simulink model "new68bus_opal"  (R2019b)
settings: Solver=ode4  StartTime=0.0  StopTime=30  FixedStep=Ts  RelTol=1e-3
PreLoadFcn:
  | PSSMODEL=1;
  | LPSS=0;
  | WAPSS=0;
  | WAPSS2=0;
  | Ts=50e-5;
InitFcn:
  | PSSMODEL=1;
  | LPSS=0;
  | WAPSS=0;
  | WAPSS2=0;
  | Ts=50e-5;
  | 
  | % Required data to 68 Bus benchmark
  | % clear
  | % clc
  | % Definition for the columns
  | % system base =100 MVA
  | 
  | %% Line data Format (line)
  | % All values are given on the same system base MVA
  | % 1: From bus
  | % 2: To bus
  | % 3: Resistance (pu)
  | % 4: Reactance  (pu)
  | % 5: Charge     (pu)
  | % 6: Transformer Tap Amplitute
  | % 7: base MVA
  | % 8: Nomonal Voltage (KV)
  | 
  | %1   2    3        4       5       6        7      8
  | line=[...
  | 1	54	0	     0.0181	  0	      1.025     100    13.8
  | 2	58	0	     0.025	  0	      1.070     100    13.8
  | 3	62	0	     0.02	  0	      1.070     100    13.8
  | 4	19	0.0007	 0.0142	  0	      1.070     100    13.8
  | 5	20	0.0009	 0.018	  0	      1.009     100    13.8
  | 6	22	0	     0.0143	  0	      1.025     100    13.8
  | 7	23	0.0005	 0.0272	  0	      0         100    13.8
  | 8	25	0.0006	 0.0232	  0	      1.025     100    13.8
  | 9	29	0.0008	 0.0156   0	      1.025     100    13.8
  | 10	31	0	     0.026	  0	      1.04      100    13.8
  | 11	32	0	     0.013	  0	      1.04      100    13.8
  | 12	36	0	     0.0075	  0	      1.04      100    13.8
  | 13	17	0	     0.0033	  0	      1.04      100    13.8
  | 14	41	0	     0.0015	  0	      1         100    13.8
  | 15	42	0	     0.0015	  0	      1         100    13.8
  | 16	18	0	     0.003	  0	      1         100    13.8
  | 17	36	0.0005	 0.0045	  0.32	  0         100    138
  | 17	43	0.0005	 0.0276	  0	      0         100    138
  | 18	42	0.004	 0.06	  2.25    0         100    138
  | 18	49	0.0076	 0.1141	  1.16    0	        100    138
  | 18	50	0.0012	 0.0288	  2.06	  0         100    138
  | 20	19	0.0007	 0.0138	  0       1.06	    100    138
  | 19	68	0.0016	 0.0195	  0.304	  0         100    138
  | 21	22	0.0008	 0.014	  0.2565  0	        100    138
  | 21	68	0.0008	 0.0135	  0.2548  0	        100    138
  | 22	23	0.0006	 0.0096	  0.1846  0	        100    138
  | 23	24	0.0022	 0.035	  0.361	  0         100    138
  | 24	68	0.0003	 0.0059	  0.068	  0         100    138
  | 25	26	0.0032	 0.0323	  0.531	  0         100    138
  | 25	54	0.007	 0.0086	  0.146	  0         100    138
  | 26	27	0.0014	 0.0147	  0.2396  0	        100    138
  | 26	28	0.0043	 0.0474	  0.7802  0	        100    138
  | 26	29	0.0057	 0.0625	  1.029	  0         100    138
  | 27	37	0.0013	 0.0173	  0.3216  0	        100    138
  | 27	53	0.032	 0.32	  0.41	  0         100    138
  | ... (+206 lines)
undefined symbols (not defined in the file or in its folder): D1, Delta, I, Left, Right, type, V
libraries: powerlib x359, artemis x26, sps_avr x16, powerlib_meascontrol x5, rtlab x1
(part 5 of 8)

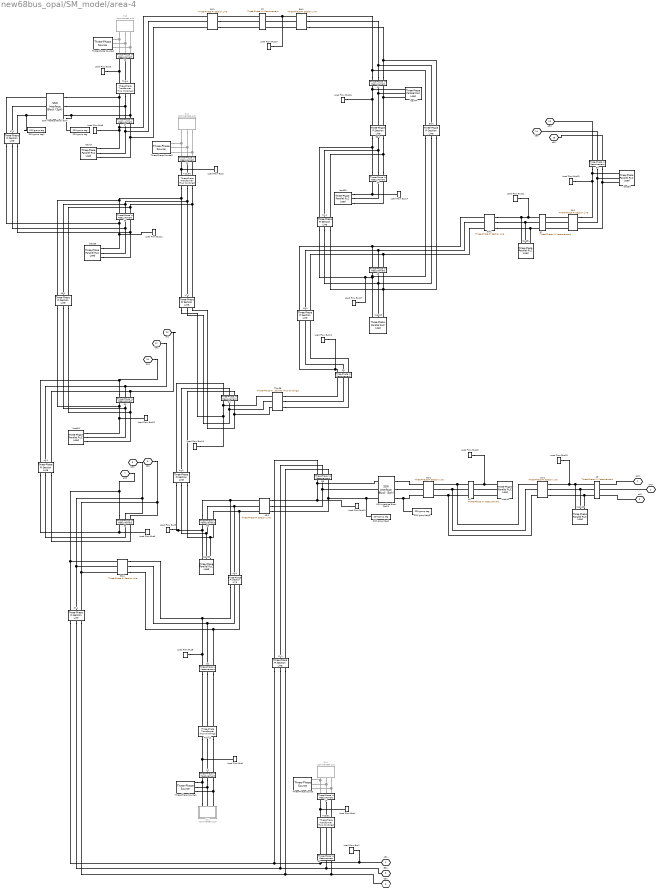
== system new68bus_opal/SM_model/area-4 ==
  10 : powerlib/Measurements/Three-Phase V-I Measurement  VoltageMeasurement=phase-to-phase  SetLabelV=on  LabelV=Vabc_10  Vpu=off  VpuLL=on  CurrentMeasurement=no  SetLabelI=off  LabelI=Iabc  Ipu=off  Pbase=100e6  Vbase=13.8e3  OutputType=Complex  PhasorSimulation=off  PSBequivalent=0
      settings: SourceProductName=Simscape Electrical
  11 : powerlib/Measurements/Three-Phase V-I Measurement  VoltageMeasurement=phase-to-phase  SetLabelV=on  LabelV=Vabc_11  Vpu=off  VpuLL=on  CurrentMeasurement=no  SetLabelI=off  LabelI=Iabc  Ipu=off  Pbase=100e6  Vbase=13.8e3  OutputType=Complex  PhasorSimulation=off  PSBequivalent=0
      settings: SourceProductName=Simscape Electrical
  12 : powerlib/Measurements/Three-Phase V-I Measurement  VoltageMeasurement=phase-to-phase  SetLabelV=on  LabelV=Vabc_12  Vpu=off  VpuLL=on  CurrentMeasurement=no  SetLabelI=off  LabelI=Iabc  Ipu=off  Pbase=100e6  Vbase=13.8e3  OutputType=Complex  PhasorSimulation=off  PSBequivalent=0
      settings: SourceProductName=Simscape Electrical
  13 : powerlib/Measurements/Three-Phase V-I Measurement  VoltageMeasurement=phase-to-phase  SetLabelV=on  LabelV=Vabc_13  Vpu=off  VpuLL=on  CurrentMeasurement=no  SetLabelI=off  LabelI=Iabc  Ipu=off  Pbase=100e6  Vbase=13.8e3  OutputType=Complex  PhasorSimulation=off  PSBequivalent=0
      settings: SourceProductName=Simscape Electrical
  17 : powerlib/Measurements/Three-Phase V-I Measurement  VoltageMeasurement=phase-to-phase  SetLabelV=on  LabelV=Vabc_17  Vpu=off  VpuLL=on  CurrentMeasurement=no  SetLabelI=off  LabelI=Iabc  Ipu=off  Pbase=100e6  Vbase=Bus(17,2)*1e3  OutputType=Complex  PhasorSimulation=off  PSBequivalent=0
      settings: SourceProductName=Simscape Electrical
  17-1 : powerlib/Elements/Three-Phase PI Section Line  LConnTagsString=a|b|c  RConnTagsString=A|B|C  Frequency=60  Resistances=[line(17,3) 3*line(17,3)]  Inductances=[line(17,4) 3*line(17,4)]  Capacitances=[line(17,5) line(17,5)/3]  Length=1
      settings: SourceProductName=Simscape Electrical
  18-1 : powerlib/Elements/Three-Phase PI Section Line  LConnTagsString=a|b|c  RConnTagsString=A|B|C  Frequency=60  Resistances=[line(18,3) 3*line(18,3)]  Inductances=[line(18,4) 3*line(18,4)]  Capacitances=[line(28,5) line(28,5)/3]  Length=1
      settings: SourceProductName=Simscape Electrical
  30 : powerlib/Measurements/Three-Phase V-I Measurement  VoltageMeasurement=phase-to-phase  SetLabelV=on  LabelV=Vabc_30  Vpu=off  VpuLL=on  CurrentMeasurement=no  SetLabelI=off  LabelI=Iabc  Ipu=off  Pbase=100e6  Vbase=Bus(30,2)*1e3  OutputType=Complex  PhasorSimulation=off  PSBequivalent=0
      settings: SourceProductName=Simscape Electrical
  31 : powerlib/Measurements/Three-Phase V-I Measurement  VoltageMeasurement=phase-to-phase  SetLabelV=on  LabelV=Vabc_31  Vpu=off  VpuLL=on  CurrentMeasurement=no  SetLabelI=off  LabelI=Iabc  Ipu=off  Pbase=100e6  Vbase=Bus(31,2)*1e3  OutputType=Complex  PhasorSimulation=off  PSBequivalent=0
      settings: SourceProductName=Simscape Electrical
  32 : powerlib/Measurements/Three-Phase V-I Measurement  VoltageMeasurement=phase-to-phase  SetLabelV=on  LabelV=Vabc_32  Vpu=off  VpuLL=on  CurrentMeasurement=no  SetLabelI=off  LabelI=Iabc  Ipu=off  Pbase=100e6  Vbase=Bus(32,2)*1e3  OutputType=Complex  PhasorSimulation=off  PSBequivalent=0
      settings: SourceProductName=Simscape Electrical
  33 : powerlib/Measurements/Three-Phase V-I Measurement  VoltageMeasurement=phase-to-phase  SetLabelV=on  LabelV=Vabc_33  Vpu=off  VpuLL=on  CurrentMeasurement=no  SetLabelI=off  LabelI=Iabc  Ipu=off  Pbase=100e6  Vbase=Bus(33,2)*1e3  OutputType=Complex  PhasorSimulation=off  PSBequivalent=0
      settings: SourceProductName=Simscape Electrical
  34 : powerlib/Measurements/Three-Phase V-I Measurement  VoltageMeasurement=phase-to-phase  SetLabelV=on  LabelV=Vabc_34  Vpu=off  VpuLL=on  CurrentMeasurement=no  SetLabelI=off  LabelI=Iabc  Ipu=off  Pbase=100e6  Vbase=Bus(34,2)*1e3  OutputType=Complex  PhasorSimulation=off  PSBequivalent=0
      settings: SourceProductName=Simscape Electrical
  35 : powerlib/Measurements/Three-Phase V-I Measurement  VoltageMeasurement=phase-to-phase  SetLabelV=on  LabelV=Vabc_35  Vpu=off  VpuLL=on  CurrentMeasurement=no  SetLabelI=off  LabelI=Iabc  Ipu=off  Pbase=100e6  Vbase=Bus(35,2)*1e3  OutputType=Complex  PhasorSimulation=off  PSBequivalent=0
      settings: SourceProductName=Simscape Electrical
  36 : powerlib/Measurements/Three-Phase V-I Measurement  VoltageMeasurement=phase-to-phase  SetLabelV=on  LabelV=Vabc_36  Vpu=off  VpuLL=on  CurrentMeasurement=no  SetLabelI=off  LabelI=Iabc  Ipu=off  Pbase=100e6  Vbase=Bus(36,2)*1e3  OutputType=Complex  PhasorSimulation=off  PSBequivalent=0
      settings: SourceProductName=Simscape Electrical
  37-1 : powerlib/Elements/Three-Phase PI Section Line  LConnTagsString=a|b|c  RConnTagsString=A|B|C  Frequency=60  Resistances=[line(37,3) 3*line(37,3)]  Inductances=[line(37,4) 3*line(37,4)]  Capacitances=[line(37,5) line(37,5)/3]  Length=1
      settings: SourceProductName=Simscape Electrical
  38 : powerlib/Measurements/Three-Phase V-I Measurement  VoltageMeasurement=phase-to-phase  SetLabelV=on  LabelV=Vabc_38  Vpu=off  VpuLL=on  CurrentMeasurement=no  SetLabelI=off  LabelI=Iabc  Ipu=off  Pbase=100e6  Vbase=Bus(38,2)*1e3  OutputType=Complex  PhasorSimulation=off  PSBequivalent=0
      settings: SourceProductName=Simscape Electrical
  38-1 : powerlib/Elements/Three-Phase PI Section Line  LConnTagsString=a|b|c  RConnTagsString=A|B|C  Frequency=60  Resistances=[line(38,3) 3*line(38,3)]  Inductances=[line(38,4) 3*line(38,4)]  Capacitances=[line(38,5) line(38,5)/3]  Length=1
      settings: SourceProductName=Simscape Electrical
  39 : powerlib/Measurements/Three-Phase V-I Measurement  VoltageMeasurement=phase-to-phase  SetLabelV=on  LabelV=Vabc_39  Vpu=off  VpuLL=on  CurrentMeasurement=no  SetLabelI=off  LabelI=Iabc  Ipu=off  Pbase=100e6  Vbase=Bus(39,2)*1e3  OutputType=Complex  PhasorSimulation=off  PSBequivalent=0
      settings: SourceProductName=Simscape Electrical
  40-1 : powerlib/Elements/Three-Phase PI Section Line  LConnTagsString=a|b|c  RConnTagsString=A|B|C  Frequency=60  Resistances=[line(40,3) 3*line(40,3)]  Inductances=[line(40,4) 3*line(40,4)]  Capacitances=[line(40,5) line(40,5)/3]  Length=1
      settings: SourceProductName=Simscape Electrical
  41-1 : powerlib/Elements/Three-Phase PI Section Line  LConnTagsString=a|b|c  RConnTagsString=A|B|C  Frequency=60  Resistances=[line(45,3) 3*line(45,3)]  Inductances=[line(45,4) 3*line(45,4)]  Capacitances=[line(45,5) line(45,5)/3]  Length=1
      settings: SourceProductName=Simscape Electrical
  43 : powerlib/Measurements/Three-Phase V-I Measurement  VoltageMeasurement=phase-to-phase  SetLabelV=on  LabelV=Vabc_43  Vpu=off  VpuLL=on  CurrentMeasurement=no  SetLabelI=off  LabelI=Iabc  Ipu=off  Pbase=100e6  Vbase=Bus(43,2)*1e3  OutputType=Complex  PhasorSimulation=off  PSBequivalent=0
      settings: SourceProductName=Simscape Electrical
  43-1 : powerlib/Elements/Three-Phase PI Section Line  LConnTagsString=a|b|c  RConnTagsString=A|B|C  Frequency=60  Resistances=[line(43,3) 3*line(43,3)]  Inductances=[line(43,4) 3*line(43,4)]  Capacitances=[line(43,5) line(43,5)/3]  Length=1
      settings: SourceProductName=Simscape Electrical
  44 : powerlib/Measurements/Three-Phase V-I Measurement  VoltageMeasurement=phase-to-phase  SetLabelV=on  LabelV=Vabc_44  Vpu=off  VpuLL=on  CurrentMeasurement=no  SetLabelI=off  LabelI=Iabc  Ipu=off  Pbase=100e6  Vbase=Bus(44,2)*1e3  OutputType=Complex  PhasorSimulation=off  PSBequivalent=0
      settings: SourceProductName=Simscape Electrical
  44-1 : powerlib/Elements/Three-Phase PI Section Line  LConnTagsString=a|b|c  RConnTagsString=A|B|C  Frequency=60  Resistances=[line(44,3) 3*line(44,3)]  Inductances=[line(44,4) 3*line(44,4)]  Capacitances=[line(44,5) line(44,5)/3]  Length=1
      settings: SourceProductName=Simscape Electrical
  45 : powerlib/Measurements/Three-Phase V-I Measurement  VoltageMeasurement=phase-to-phase  SetLabelV=on  LabelV=Vabc_45  Vpu=off  VpuLL=on  CurrentMeasurement=no  SetLabelI=off  LabelI=Iabc  Ipu=off  Pbase=100e6  Vbase=Bus(45,2)*1e3  OutputType=Complex  PhasorSimulation=off  PSBequivalent=0
      settings: SourceProductName=Simscape Electrical
  45-1 : powerlib/Elements/Three-Phase PI Section Line  LConnTagsString=a|b|c  RConnTagsString=A|B|C  Frequency=60  Resistances=[line(45,3) 3*line(45,3)]  Inductances=[line(45,4) 3*line(45,4)]  Capacitances=[line(45,5) line(45,5)/3]  Length=1
      settings: SourceProductName=Simscape Electrical
  46 : powerlib/Measurements/Three-Phase V-I Measurement  VoltageMeasurement=phase-to-phase  SetLabelV=on  LabelV=Vabc_46  Vpu=off  VpuLL=on  CurrentMeasurement=no  SetLabelI=off  LabelI=Iabc  Ipu=off  Pbase=100e6  Vbase=Bus(46,2)*1e3  OutputType=Complex  PhasorSimulation=off  PSBequivalent=0
      settings: SourceProductName=Simscape Electrical
  47-1 : powerlib/Elements/Three-Phase PI Section Line  LConnTagsString=a|b|c  RConnTagsString=A|B|C  Frequency=60  Resistances=[line(47,3) 3*line(47,3)]  Inductances=[line(47,4) 3*line(47,4)]  Capacitances=[line(47,5) line(47,5)/3]  Length=1
      settings: SourceProductName=Simscape Electrical
  48-1 : powerlib/Elements/Three-Phase PI Section Line  LConnTagsString=a|b|c  RConnTagsString=A|B|C  Frequency=60  Resistances=[line(48,3) 3*line(48,3)]  Inductances=[line(48,4) 3*line(48,4)]  Capacitances=[line(48,5) line(48,5)/3]  Length=1
      settings: SourceProductName=Simscape Electrical
  49 : powerlib/Measurements/Three-Phase V-I Measurement  VoltageMeasurement=phase-to-phase  SetLabelV=on  LabelV=Vabc_49  Vpu=off  VpuLL=on  CurrentMeasurement=no  SetLabelI=off  LabelI=Iabc  Ipu=off  Pbase=100e6  Vbase=Bus(49,2)*1e3  OutputType=Complex  PhasorSimulation=off  PSBequivalent=0
      settings: SourceProductName=Simscape Electrical
  49-1 : powerlib/Elements/Three-Phase PI Section Line  LConnTagsString=a|b|c  RConnTagsString=A|B|C  Frequency=60  Resistances=[line(49,3) 3*line(49,3)]  Inductances=[line(49,4) 3*line(49,4)]  Capacitances=[line(49,5) line(49,5)/3]  Length=1
      settings: SourceProductName=Simscape Electrical
  50 : powerlib/Measurements/Three-Phase V-I Measurement  VoltageMeasurement=phase-to-phase  SetLabelV=on  LabelV=Vabc_50  Vpu=off  VpuLL=on  CurrentMeasurement=no  SetLabelI=off  LabelI=Iabc  Ipu=off  Pbase=100e6  Vbase=Bus(50,2)*1e3  OutputType=Complex  PhasorSimulation=off  PSBequivalent=0
      settings: SourceProductName=Simscape Electrical
  51 : powerlib/Measurements/Three-Phase V-I Measurement  VoltageMeasurement=phase-to-phase  SetLabelV=on  LabelV=Vabc_51  Vpu=off  VpuLL=on  CurrentMeasurement=no  SetLabelI=off  LabelI=Iabc  Ipu=off  Pbase=100e6  Vbase=Bus(51,2)*1e3  OutputType=Complex  PhasorSimulation=off  PSBequivalent=0
      settings: SourceProductName=Simscape Electrical
  52-1 : powerlib/Elements/Three-Phase PI Section Line  LConnTagsString=a|b|c  RConnTagsString=A|B|C  Frequency=60  Resistances=[line(52,3) 3*line(52,3)]  Inductances=[line(52,4) 3*line(52,4)]  Capacitances=[line(52,5) line(52,5)/3]  Length=1
      settings: SourceProductName=Simscape Electrical
  53-1 : powerlib/Elements/Three-Phase PI Section Line  LConnTagsString=a|b|c  RConnTagsString=A|B|C  Frequency=60  Resistances=[line(52,4) 3*line(52,4)]  Inductances=[line(53,4) 3*line(53,4)]  Capacitances=[line(28,5) line(28,5)/3]  Length=1
      settings: SourceProductName=Simscape Electrical
  54-1 : powerlib/Elements/Three-Phase PI Section Line  LConnTagsString=a|b|c  RConnTagsString=A|B|C  Frequency=60  Resistances=[line(52,4) 3*line(52,4)]  Inductances=[line(54,4) 3*line(54,4)]  Capacitances=[line(28,5) line(28,5)/3]  Length=1
      settings: SourceProductName=Simscape Electrical
  58-1 : powerlib/Elements/Three-Phase PI Section Line  LConnTagsString=a|b|c  RConnTagsString=A|B|C  Frequency=60  Resistances=[line(58,3) 3*line(58,3)]  Inductances=[line(58,4) 3*line(58,4)]  Capacitances=[line(28,5) line(28,5)/3]  Length=1
      settings: SourceProductName=Simscape Electrical
  59-1 : powerlib/Elements/Three-Phase PI Section Line  LConnTagsString=a|b|c  RConnTagsString=A|B|C  Frequency=60  Resistances=[line(59,3) 3*line(59,3)]  Inductances=[line(59,4) 3*line(59,4)]  Capacitances=[line(28,5) line(28,5)/3]  Length=1
      settings: SourceProductName=Simscape Electrical
  60-1 : powerlib/Elements/Three-Phase PI Section Line  LConnTagsString=a|b|c  RConnTagsString=A|B|C  Frequency=60  Resistances=[line(60,3) 3*line(60,3)]  Inductances=[line(60,4) 3*line(60,4)]  Capacitances=[line(60,5) line(60,5)/3]  Length=1
      settings: SourceProductName=Simscape Electrical
  61 : powerlib/Measurements/Three-Phase V-I Measurement  VoltageMeasurement=phase-to-phase  SetLabelV=on  LabelV=Vabc_61  Vpu=off  VpuLL=on  CurrentMeasurement=no  SetLabelI=off  LabelI=Iabc  Ipu=off  Pbase=100e6  Vbase=Bus(61,2)*1e3  OutputType=Complex  PhasorSimulation=off  PSBequivalent=0
      settings: SourceProductName=Simscape Electrical
  61-1 : powerlib/Elements/Three-Phase PI Section Line  LConnTagsString=a|b|c  RConnTagsString=A|B|C  Frequency=60  Resistances=[line(61,3) 3*line(61,3)]  Inductances=[line(61,4) 3*line(61,4)]  Capacitances=[line(61,5) line(61,5)/3]  Length=1
      settings: SourceProductName=Simscape Electrical
  64-1 : powerlib/Elements/Three-Phase PI Section Line  LConnTagsString=a|b|c  RConnTagsString=A|B|C  Frequency=60  Resistances=[line(64,3) 3*line(64,3)]  Inductances=[line(64,4) 3*line(64,4)]  Capacitances=[line(64,5) line(64,5)/3]  Length=1
      settings: SourceProductName=Simscape Electrical
  G10 : Subsystem  Commented=on
  G11 : Subsystem  Commented=on
  G12 : Subsystem  Commented=on
  G13 : Subsystem  Commented=on
  Load Flow Bus1 : powerlib/Measurements/Load Flow Bus  LConnTagsString=a  Phases=single  Connectors=on one side  ID=BUS_11  Vbase=13.8e3  Vref=1  Vangle=0  VLF=1  VLFb=1  VLFc=1  angleLF=0  angleLFb=0  angleLFc=0
      settings: SourceProductName=Simscape Electrical
  Load Flow Bus10 : powerlib/Measurements/Load Flow Bus  LConnTagsString=a  Phases=single  Connectors=on one side  ID=BUS_34  Vbase=138e3  Vref=1  Vangle=0  VLF=1  VLFb=1  VLFc=1  angleLF=0  angleLFb=0  angleLFc=0
      settings: SourceProductName=Simscape Electrical
  Load Flow Bus11 : powerlib/Measurements/Load Flow Bus  LConnTagsString=a  Phases=single  Connectors=on one side  ID=BUS_35  Vbase=138e3  Vref=1  Vangle=0  VLF=1  VLFb=1  VLFc=1  angleLF=0  angleLFb=0  angleLFc=0
      settings: SourceProductName=Simscape Electrical
  Load Flow Bus12 : powerlib/Measurements/Load Flow Bus  LConnTagsString=a  Phases=single  Connectors=on one side  ID=BUS_36  Vbase=138e3  Vref=1  Vangle=0  VLF=1  VLFb=1  VLFc=1  angleLF=0  angleLFb=0  angleLFc=0
      settings: SourceProductName=Simscape Electrical
  Load Flow Bus13 : powerlib/Measurements/Load Flow Bus  LConnTagsString=a  Phases=single  Connectors=on one side  ID=BUS_38  Vbase=138e3  Vref=1  Vangle=0  VLF=1  VLFb=1  VLFc=1  angleLF=0  angleLFb=0  angleLFc=0
      settings: SourceProductName=Simscape Electrical
  Load Flow Bus14 : powerlib/Measurements/Load Flow Bus  LConnTagsString=a  Phases=single  Connectors=on one side  ID=BUS_39  Vbase=138e3  Vref=1  Vangle=0  VLF=1  VLFb=1  VLFc=1  angleLF=0  angleLFb=0  angleLFc=0
      settings: SourceProductName=Simscape Electrical
  Load Flow Bus15 : powerlib/Measurements/Load Flow Bus  LConnTagsString=a  Phases=single  Connectors=on one side  ID=BUS_43  Vbase=138e3  Vref=1  Vangle=0  VLF=1  VLFb=1  VLFc=1  angleLF=0  angleLFb=0  angleLFc=0
      settings: SourceProductName=Simscape Electrical
  Load Flow Bus16 : powerlib/Measurements/Load Flow Bus  LConnTagsString=a  Phases=single  Connectors=on one side  ID=BUS_44  Vbase=138e3  Vref=1  Vangle=0  VLF=1  VLFb=1  VLFc=1  angleLF=0  angleLFb=0  angleLFc=0
      settings: SourceProductName=Simscape Electrical
  Load Flow Bus17 : powerlib/Measurements/Load Flow Bus  LConnTagsString=a  Phases=single  Connectors=on one side  ID=BUS_45  Vbase=138e3  Vref=1  Vangle=0  VLF=1  VLFb=1  VLFc=1  angleLF=0  angleLFb=0  angleLFc=0
      settings: SourceProductName=Simscape Electrical
  Load Flow Bus18 : powerlib/Measurements/Load Flow Bus  LConnTagsString=a  Phases=single  Connectors=on one side  ID=BUS_46  Vbase=138e3  Vref=1  Vangle=0  VLF=1  VLFb=1  VLFc=1  angleLF=0  angleLFb=0  angleLFc=0
      settings: SourceProductName=Simscape Electrical
  Load Flow Bus19 : powerlib/Measurements/Load Flow Bus  LConnTagsString=a  Phases=single  Connectors=on one side  ID=BUS_49  Vbase=138e3  Vref=1  Vangle=0  VLF=1  VLFb=1  VLFc=1  angleLF=0  angleLFb=0  angleLFc=0
      settings: SourceProductName=Simscape Electrical
  Load Flow Bus2 : powerlib/Measurements/Load Flow Bus  LConnTagsString=a  Phases=single  Connectors=on one side  ID=BUS_12  Vbase=13.8e3  Vref=1.0156  Vangle=0  VLF=1  VLFb=1  VLFc=1  angleLF=0  angleLFb=0  angleLFc=0
      settings: SourceProductName=Simscape Electrical
  Load Flow Bus20 : powerlib/Measurements/Load Flow Bus  LConnTagsString=a  Phases=single  Connectors=on one side  ID=BUS_50  Vbase=138e3  Vref=1  Vangle=0  VLF=1  VLFb=1  VLFc=1  angleLF=0  angleLFb=0  angleLFc=0
      settings: SourceProductName=Simscape Electrical
  Load Flow Bus21 : powerlib/Measurements/Load Flow Bus  LConnTagsString=a  Phases=single  Connectors=on one side  ID=BUS_51  Vbase=138e3  Vref=1  Vangle=0  VLF=1  VLFb=1  VLFc=1  angleLF=0  angleLFb=0  angleLFc=0
      settings: SourceProductName=Simscape Electrical
  Load Flow Bus22 : powerlib/Measurements/Load Flow Bus  LConnTagsString=a  Phases=single  Connectors=on one side  ID=BUS_61  Vbase=138e3  Vref=1  Vangle=0  VLF=1  VLFb=1  VLFc=1  angleLF=0  angleLFb=0  angleLFc=0
      settings: SourceProductName=Simscape Electrical
  Load Flow Bus3 : powerlib/Measurements/Load Flow Bus  LConnTagsString=a  Phases=single  Connectors=on one side  ID=BUS_13  Vbase=13.8e3  Vref=1.011  Vangle=0  VLF=1  VLFb=1  VLFc=1  angleLF=0  angleLFb=0  angleLFc=0
      settings: SourceProductName=Simscape Electrical
  Load Flow Bus4 : powerlib/Measurements/Load Flow Bus  LConnTagsString=a  Phases=single  Connectors=on one side  ID=BUS_10  Vbase=13.8e3  Vref=1.01  Vangle=0  VLF=1  VLFb=1  VLFc=1  angleLF=0  angleLFb=0  angleLFc=0
      settings: SourceProductName=Simscape Electrical
  Load Flow Bus5 : powerlib/Measurements/Load Flow Bus  LConnTagsString=a  Phases=single  Connectors=on one side  ID=BUS_17  Vbase=138e3  Vref=1  Vangle=0  VLF=1  VLFb=1  VLFc=1  angleLF=0  angleLFb=0  angleLFc=0
      settings: SourceProductName=Simscape Electrical
  Load Flow Bus6 : powerlib/Measurements/Load Flow Bus  LConnTagsString=a  Phases=single  Connectors=on one side  ID=BUS_30  Vbase=138e3  Vref=1  Vangle=0  VLF=1  VLFb=1  VLFc=1  angleLF=0  angleLFb=0  angleLFc=0
      settings: SourceProductName=Simscape Electrical
  Load Flow Bus7 : powerlib/Measurements/Load Flow Bus  LConnTagsString=a  Phases=single  Connectors=on one side  ID=BUS_31  Vbase=138e3  Vref=1  Vangle=0  VLF=1  VLFb=1  VLFc=1  angleLF=0  angleLFb=0  angleLFc=0
      settings: SourceProductName=Simscape Electrical
  Load Flow Bus8 : powerlib/Measurements/Load Flow Bus  LConnTagsString=a  Phases=single  Connectors=on one side  ID=BUS_32  Vbase=138e3  Vref=1  Vangle=0  VLF=1  VLFb=1  VLFc=1  angleLF=0  angleLFb=0  angleLFc=0
      settings: SourceProductName=Simscape Electrical
  Load Flow Bus9 : powerlib/Measurements/Load Flow Bus  LConnTagsString=a  Phases=single  Connectors=on one side  ID=BUS_33  Vbase=138e3  Vref=1  Vangle=0  VLF=1  VLFb=1  VLFc=1  angleLF=0  angleLFb=0  angleLFc=0
      settings: SourceProductName=Simscape Electrical
  SSN Interface Block (3ph) : artemis/SSN/Nodal Interface Blocks/SSN Interface Block (3ph)  nb_phase=3  nb_port=2  p1_type=I-type(Left)  p2_type=I-type(Right)  p3_type=V-type(Left)  p4_type=V-type(Left)  p5_type=V-type(Left)  p6_type=V-type(Left)  p7_type=V-type(Left)  p8_type=V-type(Left)  p9_type=V-type(Left)  p10_type=V-type(Left)  p11_type=V-type(Left)  p12_type=V-type(Left)  p13_type=V-type(Left)  p14_type=V-type(Left)  p15_type=V-type(Left)  p16_type=V-type(Left)  I_port_shunt_resistance=1e9
  SSN Interface Block (3ph)1 : artemis/SSN/Nodal Interface Blocks/SSN Interface Block (3ph)  nb_phase=3  nb_port=2  p1_type=I-type(Left)  p2_type=I-type(Right)  p3_type=V-type(Left)  p4_type=V-type(Left)  p5_type=V-type(Left)  p6_type=V-type(Left)  p7_type=V-type(Left)  p8_type=V-type(Left)  p9_type=V-type(Left)  p10_type=V-type(Left)  p11_type=V-type(Left)  p12_type=V-type(Left)  p13_type=V-type(Left)  p14_type=V-type(Left)  p15_type=V-type(Left)  p16_type=V-type(Left)  I_port_shunt_resistance=1e9
  SSN group tag : artemis/SSN/SSN group tag  ssn_group_tag=ssn7a
  SSN group tag1 : artemis/SSN/SSN group tag  ssn_group_tag=ssn7b
  SSN group tag2 : artemis/SSN/SSN group tag  ssn_group_tag=ssn8a
  SSN group tag3 : artemis/SSN/SSN group tag  ssn_group_tag=ssn8b
  T10-31 : powerlib/Elements/Three-Phase Transformer (Two Windings)  Winding1Connection=Delta (D1)  Winding2Connection=Yg  CoreType=Three single-phase transformers  SetSaturation=off  Hysteresis=off  DataFile='hysteresis'  SetInitialFlux=off  Measurements=None  UNITS=pu  NominalPower=[ 10000e6 , 60 ]  Winding1=[ 13.8e3 , 0.0002 , 0 ]  Winding2=[ 138e3 , 0.0002 , 0.026 ]  Rm=500  Lm=500  L0=0.5  Saturation=[ 0,0 ; 0.0024,1.2 ; 1.0,1.52 ]  InitialFluxes=[ 0.8 , -0.8 , 0.7 ]  BreakLoop=off  DiscreteSolver=Trapezoidal robust  DataType=off  TransfoNumber=1
      settings: SourceProductName=Simscape Electrical
  T12-36 : powerlib/Elements/Three-Phase Transformer (Two Windings)  Winding1Connection=Delta (D1)  Winding2Connection=Yg  CoreType=Three single-phase transformers  SetSaturation=off  Hysteresis=off  DataFile='hysteresis'  SetInitialFlux=off  Measurements=None  UNITS=pu  NominalPower=[ 10000e6 , 60 ]  Winding1=[ 13.8e3 , 0.002 , 0 ]  Winding2=[ 138e3 , 0.002 , 0.0075 ]  Rm=500  Lm=500  L0=0.5  Saturation=[ 0,0 ; 0.0024,1.2 ; 1.0,1.52 ]  InitialFluxes=[ 0.8 , -0.8 , 0.7 ]  BreakLoop=off  DiscreteSolver=Trapezoidal robust  DataType=off  TransfoNumber=1
      settings: SourceProductName=Simscape Electrical
  T13-1 : powerlib/Elements/Three-Phase Transformer (Two Windings)  Winding1Connection=Delta (D1)  Winding2Connection=Yg  CoreType=Three single-phase transformers  SetSaturation=off  Hysteresis=off  DataFile='hysteresis'  SetInitialFlux=off  Measurements=None  UNITS=pu  NominalPower=[ 10000e6 , 60 ]  Winding1=[ 13.8e3 , 0.0002 , 0 ]  Winding2=[ 138e3 , 0.0002, 0.0033 ]  Rm=500  Lm=500  L0=0.5  Saturation=[ 0,0 ; 0.0024,1.2 ; 1.0,1.52 ]  InitialFluxes=[ 0.8 , -0.8 , 0.7 ]  BreakLoop=off  DiscreteSolver=Trapezoidal robust  DataType=off  TransfoNumber=1
      settings: SourceProductName=Simscape Electrical
  T32-11 : powerlib/Elements/Three-Phase Transformer (Two Windings)  Winding1Connection=Delta (D1)  Winding2Connection=Yg  CoreType=Three single-phase transformers  SetSaturation=off  Hysteresis=off  DataFile='hysteresis'  SetInitialFlux=off  Measurements=None  UNITS=pu  NominalPower=[ 10000e6 , 60 ]  Winding1=[ 13.8e3 , 0.00020 , 0 ]  Winding2=[ 138e3 , 0.0002 , 0.013 ]  Rm=500  Lm=500  L0=0.5  Saturation=[ 0,0 ; 0.0024,1.2 ; 1.0,1.52 ]  InitialFluxes=[ 0.8 , -0.8 , 0.7 ]  BreakLoop=off  DiscreteSolver=Trapezoidal robust  DataType=off  TransfoNumber=1
      settings: SourceProductName=Simscape Electrical
  T34-35 : powerlib/Elements/Three-Phase Transformer (Two Windings)  Winding1Connection=Y  Winding2Connection=Y  CoreType=Three single-phase transformers  SetSaturation=off  Hysteresis=off  DataFile='hysteresis'  SetInitialFlux=off  Measurements=None  UNITS=pu  NominalPower=[ 10000e6 , 60 ]  Winding1=[ 138e3 , 0.00005 , 0 ]  Winding2=[ 138e3 , 0.00005 , 0.0074 ]  Rm=500  Lm=500  L0=0.5  Saturation=[ 0,0 ; 0.0024,1.2 ; 1.0,1.52 ]  InitialFluxes=[ 0.8 , -0.8 , 0.7 ]  BreakLoop=off  DiscreteSolver=Trapezoidal robust  DataType=off  TransfoNumber=1
      settings: SourceProductName=Simscape Electrical
  Three-Phase Source : powerlib/Electrical Sources/Three-Phase Source  InternalConnection=Yg  VoltagePhases=off  Voltage=13.8e3  PhaseAngle=0  Voltage_phases=[25e3 25e3 25e3]/sqrt(3)  PhaseAngles_phases=[0 -120 +120]  Frequency=60  NonIdealSource=on  SpecifyImpedance=off  Resistance=0.8929  Inductance=16.58e-3  ShortCircuitLevel=100e6  BaseVoltage=13.8e3  XRratio=7  BusType=PV  Pref=500e6  Qref=0  Prefabc=[10e3, 10e3, 10e3]  Qrefabc=[0, 0, 0]  Qmin=-inf  Qmax=inf
      settings: SourceProductName=Simscape Electrical
  Three-Phase Source1 : powerlib/Electrical Sources/Three-Phase Source  InternalConnection=Yg  VoltagePhases=off  Voltage=13.8e3  PhaseAngle=0  Voltage_phases=[25e3 25e3 25e3]/sqrt(3)  PhaseAngles_phases=[0 -120 +120]  Frequency=60  NonIdealSource=on  SpecifyImpedance=off  Resistance=0.8929  Inductance=16.58e-3  ShortCircuitLevel=100e6  BaseVoltage=13.8e3  XRratio=7  BusType=PV  Pref=1000e6  Qref=0  Prefabc=[10e3, 10e3, 10e3]  Qrefabc=[0, 0, 0]  Qmin=-inf  Qmax=inf
      settings: SourceProductName=Simscape Electrical
  Three-Phase Source2 : powerlib/Electrical Sources/Three-Phase Source  InternalConnection=Yg  VoltagePhases=off  Voltage=13.8e3*1.011  PhaseAngle=0  Voltage_phases=[25e3 25e3 25e3]/sqrt(3)  PhaseAngles_phases=[0 -120 +120]  Frequency=60  NonIdealSource=on  SpecifyImpedance=off  Resistance=0.8929  Inductance=16.58e-3  ShortCircuitLevel=100e6  BaseVoltage=13.8e3  XRratio=7  BusType=PV  Pref=3591e6  Qref=0  Prefabc=[10e3, 10e3, 10e3]  Qrefabc=[0, 0, 0]  Qmin=-inf  Qmax=inf
      settings: SourceProductName=Simscape Electrical
  Three-Phase Source3 : powerlib/Electrical Sources/Three-Phase Source  InternalConnection=Yg  VoltagePhases=off  Voltage=13.8e3*1.0156  PhaseAngle=0  Voltage_phases=[25e3 25e3 25e3]/sqrt(3)  PhaseAngles_phases=[0 -120 +120]  Frequency=60  NonIdealSource=on  SpecifyImpedance=off  Resistance=0.8929  Inductance=16.58e-3  ShortCircuitLevel=100e6  BaseVoltage=13.8e3  XRratio=7  BusType=PV  Pref=1350e6  Qref=0  Prefabc=[10e3, 10e3, 10e3]  Qrefabc=[0, 0, 0]  Qmin=-inf  Qmax=inf
      settings: SourceProductName=Simscape Electrical
  load17 : powerlib/Elements/Three-Phase Parallel RLC Load  LConnTagsString=A|B|C  Configuration=Y (grounded)  NominalVoltage=138000  Vabc=[1e3 1e3 1e3]  Vabcp=[1e3 1e3 1e3]  NominalFrequency=60  UnbalancedPower=off  ActivePower=6000e6  InductivePower=300e6  CapacitivePower=0  Pabc=[10e3 9e3 11e3]  QLabc=[100 90 110]  QCabc=[100 90 110]  Pabcp=[10e3 9e3 11e3]  QLabcp=[100 90 110]  QCabcp=[100 90 110]  Measurements=None  LoadType=constant PQ
      settings: SourceProductName=Simscape Electrical
  load33 : powerlib/Elements/Three-Phase Parallel RLC Load  LConnTagsString=A|B|C  Configuration=Y (grounded)  NominalVoltage=138000  Vabc=[1e3 1e3 1e3]  Vabcp=[1e3 1e3 1e3]  NominalFrequency=60  UnbalancedPower=off  ActivePower=112e6  InductivePower=0  CapacitivePower=0  Pabc=[10e3 9e3 11e3]  QLabc=[100 90 110]  QCabc=[100 90 110]  Pabcp=[10e3 9e3 11e3]  QLabcp=[100 90 110]  QCabcp=[100 90 110]  Measurements=None  LoadType=constant PQ
      settings: SourceProductName=Simscape Electrical
  load36 : powerlib/Elements/Three-Phase Parallel RLC Load  LConnTagsString=A|B|C  Configuration=Y (grounded)  NominalVoltage=138000  Vabc=[1e3 1e3 1e3]  Vabcp=[1e3 1e3 1e3]  NominalFrequency=60  UnbalancedPower=off  ActivePower=102e6  InductivePower=0  CapacitivePower=19.6e6  Pabc=[10e3 9e3 11e3]  QLabc=[100 90 110]  QCabc=[100 90 110]  Pabcp=[10e3 9e3 11e3]  QLabcp=[100 90 110]  QCabcp=[100 90 110]  Measurements=None  LoadType=constant PQ
      settings: SourceProductName=Simscape Electrical
  load39 : powerlib/Elements/Three-Phase Parallel RLC Load  LConnTagsString=A|B|C  Configuration=Y (grounded)  NominalVoltage=138000  Vabc=[1e3 1e3 1e3]  Vabcp=[1e3 1e3 1e3]  NominalFrequency=60  UnbalancedPower=off  ActivePower=267e6  InductivePower=13e6  CapacitivePower=0  Pabc=[10e3 9e3 11e3]  QLabc=[100 90 110]  QCabc=[100 90 110]  Pabcp=[10e3 9e3 11e3]  QLabcp=[100 90 110]  QCabcp=[100 90 110]  Measurements=None  LoadType=constant PQ
      settings: SourceProductName=Simscape Electrical
  load44 : powerlib/Elements/Three-Phase Parallel RLC Load  LConnTagsString=A|B|C  Configuration=Y (grounded)  NominalVoltage=138000  Vabc=[1e3 1e3 1e3]  Vabcp=[1e3 1e3 1e3]  NominalFrequency=60  UnbalancedPower=off  ActivePower=268e6  InductivePower=5e6  CapacitivePower=0  Pabc=[10e3 9e3 11e3]  QLabc=[100 90 110]  QCabc=[100 90 110]  Pabcp=[10e3 9e3 11e3]  QLabcp=[100 90 110]  QCabcp=[100 90 110]  Measurements=None  LoadType=constant PQ
      settings: SourceProductName=Simscape Electrical
  load45 : powerlib/Elements/Three-Phase Parallel RLC Load  LConnTagsString=A|B|C  Configuration=Y (grounded)  NominalVoltage=138000  Vabc=[1e3 1e3 1e3]  Vabcp=[1e3 1e3 1e3]  NominalFrequency=60  UnbalancedPower=off  ActivePower=208e6  InductivePower=21e06  CapacitivePower=0  Pabc=[10e3 9e3 11e3]  QLabc=[100 90 110]  QCabc=[100 90 110]  Pabcp=[10e3 9e3 11e3]  QLabcp=[100 90 110]  QCabcp=[100 90 110]  Measurements=None  LoadType=constant PQ
      settings: SourceProductName=Simscape Electrical
  load46 : powerlib/Elements/Three-Phase Parallel RLC Load  LConnTagsString=A|B|C  Configuration=Y (grounded)  NominalVoltage=138000  Vabc=[1e3 1e3 1e3]  Vabcp=[1e3 1e3 1e3]  NominalFrequency=60  UnbalancedPower=off  ActivePower=151e6  InductivePower=28e6  CapacitivePower=0  Pabc=[10e3 9e3 11e3]  QLabc=[100 90 110]  QCabc=[100 90 110]  Pabcp=[10e3 9e3 11e3]  QLabcp=[100 90 110]  QCabcp=[100 90 110]  Measurements=None  LoadType=constant PQ
      settings: SourceProductName=Simscape Electrical
  load49 : powerlib/Elements/Three-Phase Parallel RLC Load  LConnTagsString=A|B|C  Configuration=Y (grounded)  NominalVoltage=138000  Vabc=[1e3 1e3 1e3]  Vabcp=[1e3 1e3 1e3]  NominalFrequency=60  UnbalancedPower=off  ActivePower=164e6  InductivePower=29e6  CapacitivePower=0  Pabc=[10e3 9e3 11e3]  QLabc=[100 90 110]  QCabc=[100 90 110]  Pabcp=[10e3 9e3 11e3]  QLabcp=[100 90 110]  QCabcp=[100 90 110]  Measurements=None  LoadType=constant PQ
      settings: SourceProductName=Simscape Electrical
  load50 : powerlib/Elements/Three-Phase Parallel RLC Load  LConnTagsString=A|B|C  Configuration=Y (grounded)  NominalVoltage=138000  Vabc=[1e3 1e3 1e3]  Vabcp=[1e3 1e3 1e3]  NominalFrequency=60  UnbalancedPower=off  ActivePower=100e6  InductivePower=0  CapacitivePower=147e06  Pabc=[10e3 9e3 11e3]  QLabc=[100 90 110]  QCabc=[100 90 110]  Pabcp=[10e3 9e3 11e3]  QLabcp=[100 90 110]  QCabcp=[100 90 110]  Measurements=None  LoadType=constant PQ
      settings: SourceProductName=Simscape Electrical
  load51 : powerlib/Elements/Three-Phase Parallel RLC Load  LConnTagsString=A|B|C  Configuration=Y (grounded)  NominalVoltage=138000  Vabc=[1e3 1e3 1e3]  Vabcp=[1e3 1e3 1e3]  NominalFrequency=60  UnbalancedPower=off  ActivePower=337e6  InductivePower=0  CapacitivePower=122e06  Pabc=[10e3 9e3 11e3]  QLabc=[100 90 110]  QCabc=[100 90 110]  Pabcp=[10e3 9e3 11e3]  QLabcp=[100 90 110]  QCabcp=[100 90 110]  Measurements=None  LoadType=constant PQ
      settings: SourceProductName=Simscape Electrical
  load61 : powerlib/Elements/Three-Phase Parallel RLC Load  LConnTagsString=A|B|C  Configuration=Y (grounded)  NominalVoltage=138000  Vabc=[1e3 1e3 1e3]  Vabcp=[1e3 1e3 1e3]  NominalFrequency=60  UnbalancedPower=off  ActivePower=104e6  InductivePower=125e6  CapacitivePower=0  Pabc=[10e3 9e3 11e3]  QLabc=[100 90 110]  QCabc=[100 90 110]  Pabcp=[10e3 9e3 11e3]  QLabcp=[100 90 110]  QCabcp=[100 90 110]  Measurements=None  LoadType=constant PQ
      settings: SourceProductName=Simscape Electrical
  a49 : PMIOPort  Tag=PMCPort  Side=Right
  b49 : PMIOPort  Tag=PMCPort  Port=2  Side=Right
  c49 : PMIOPort  Tag=PMCPort  Port=3  Side=Right
  A31 : PMIOPort  Tag=PMCPort  Port=4  Side=Right
  B31 : PMIOPort  Tag=PMCPort  Port=5  Side=Right
  C31 : PMIOPort  Tag=PMCPort  Port=6  Side=Right
  a30 : PMIOPort  Tag=PMCPort  Port=7  Side=Right
  b30 : PMIOPort  Tag=PMCPort  Port=8  Side=Right
  c30 : PMIOPort  Tag=PMCPort  Port=9  Side=Right
  a61 : PMIOPort  Tag=PMCPort  Port=10  Side=Right
  b61 : PMIOPort  Tag=PMCPort  Port=11  Side=Right
  c61 : PMIOPort  Tag=PMCPort  Port=12  Side=Right
  a50 : PMIOPort  Tag=PMCPort  Port=13  Side=Right
  b50 : PMIOPort  Tag=PMCPort  Port=14  Side=Right
  c50 : PMIOPort  Tag=PMCPort  Port=15  Side=Right
  connections:
  G13/LConn1 -- Three-Phase Source2/RConn1 -- 13/RConn1
  T13-1/LConn1 -- 13/LConn1 -- Load Flow Bus3/LConn1
  T13-1/RConn2 -- SSN Interface Block (3ph)/LConn2 -- 17/RConn2
  G13/LConn3 -- Three-Phase Source2/RConn3 -- 13/RConn3
  G13/LConn2 -- Three-Phase Source2/RConn2 -- 13/RConn2
  17/RConn3 -- SSN group tag/LConn1 -- SSN Interface Block (3ph)/LConn3 -- T13-1/RConn3
  T13-1/RConn1 -- SSN Interface Block (3ph)/LConn1 -- 17/RConn1
  load17/LConn1 -- Load Flow Bus5/LConn1 -- 17/LConn1 -- 18-1/RConn1
  load17/LConn2 -- 17/LConn2 -- 18-1/RConn2
  load17/LConn3 -- 18-1/RConn3 -- 17/LConn3
  49-1/LConn1 -- 36/RConn1 -- 47-1/LConn1 -- T12-36/RConn1
  T12-36/RConn2 -- 49-1/LConn2 -- 36/RConn2 -- 47-1/LConn2
  T12-36/RConn3 -- 49-1/LConn3 -- 36/RConn3 -- 47-1/LConn3
  G12/LConn1 -- Three-Phase Source3/RConn1 -- 12/RConn1
  G12/LConn2 -- Three-Phase Source3/RConn2 -- 12/RConn2
  G12/LConn3 -- Three-Phase Source3/RConn3 -- 12/RConn3
  T12-36/LConn1 -- Load Flow Bus2/LConn1 -- 12/LConn1
  T12-36/LConn2 -- 12/LConn2
  T12-36/LConn3 -- 12/LConn3
  load36/LConn1 -- Load Flow Bus12/LConn1 -- 17-1/RConn1 -- 36/LConn1
  load36/LConn2 -- 17-1/RConn2 -- 36/LConn2
  load36/LConn3 -- 17-1/RConn3 -- 36/LConn3
  61/RConn1 -- a61/RConn1 -- 40-1/LConn1
  b61/RConn1 -- 61/RConn2 -- 40-1/LConn2
  c61/RConn1 -- 61/RConn3 -- 40-1/LConn3
  load61/LConn1 -- Load Flow Bus22/LConn1 -- 61/LConn1 -- 49-1/RConn1
  load61/LConn2 -- 61/LConn2 -- 49-1/RConn2
  load61/LConn3 -- 61/LConn3 -- 49-1/RConn3
  30/RConn1 -- a30/RConn1 -- 38-1/LConn1 -- 37-1/LConn1
  37-1/LConn2 -- 30/RConn2 -- b30/RConn1 -- 38-1/LConn2
  37-1/LConn3 -- 30/RConn3 -- c30/RConn1 -- 38-1/LConn3
  47-1/RConn1 -- 34/LConn1 -- T34-35/LConn1 -- Load Flow Bus10/LConn1
  47-1/RConn2 -- T34-35/LConn2 -- 34/LConn2
  47-1/RConn3 -- T34-35/LConn3 -- 34/LConn3
  33/RConn1 -- 45-1/LConn1 -- 43-1/LConn1
  45-1/LConn2 -- 33/RConn2 -- 43-1/LConn2
  45-1/LConn3 -- 33/RConn3 -- 43-1/LConn3
  44-1/RConn1 -- Load Flow Bus9/LConn1 -- 33/LConn1 -- load33/LConn1
  load33/LConn2 -- 44-1/RConn2 -- 33/LConn2
  33/LConn3 -- 44-1/RConn3 -- load33/LConn3
  38-1/RConn1 -- Load Flow Bus8/LConn1 -- 32/LConn1 -- 43-1/RConn1
  32/LConn2 -- 38-1/RConn2 -- 43-1/RConn2
  32/LConn3 -- 38-1/RConn3 -- 43-1/RConn3
  40-1/RConn1 -- Load Flow Bus6/LConn1 -- 30/LConn1
  40-1/RConn2 -- 30/LConn2
  40-1/RConn3 -- 30/LConn3
  G11/LConn1 -- Three-Phase Source1/RConn1 -- 11/RConn1
  45-1/RConn1 -- Load Flow Bus13/LConn1 -- SSN Interface Block (3ph)1/LConn1 -- 38/LConn1
  45-1/RConn2 -- SSN Interface Block (3ph)1/LConn2 -- 38/LConn2
  45-1/RConn3 -- SSN group tag2/LConn1 -- SSN Interface Block (3ph)1/LConn3 -- 38/LConn3
  G10/LConn1 -- 10/RConn1 -- Three-Phase Source/RConn1
  G10/LConn2 -- Three-Phase Source/RConn2 -- 10/RConn2
  G10/LConn3 -- Three-Phase Source/RConn3 -- 10/RConn3
  T10-31/LConn1 -- Load Flow Bus4/LConn1 -- 10/LConn1
  T10-31/LConn2 -- 10/LConn2
  T10-31/LConn3 -- 10/LConn3
  31/RConn1 -- T10-31/RConn1
  31/RConn2 -- T10-31/RConn2
  31/RConn3 -- T10-31/RConn3
  41-1/LConn1 -- 38/RConn1
  41-1/LConn2 -- 38/RConn2
  41-1/LConn3 -- 38/RConn3
  43/RConn1 -- 18-1/LConn1
  18-1/LConn2 -- 43/RConn2
  18-1/LConn3 -- 43/RConn3
  58-1/RConn1 -- Load Flow Bus15/LConn1 -- 43/LConn1
  58-1/RConn2 -- 43/LConn2
  58-1/RConn3 -- 43/LConn3
  44/RConn1 -- 58-1/LConn1 -- 59-1/LConn1
  44/RConn2 -- 58-1/LConn2 -- 59-1/LConn2
  44/RConn3 -- 58-1/LConn3 -- 59-1/LConn3
  53-1/RConn1 -- Load Flow Bus16/LConn1 -- load44/LConn1 -- 44/LConn1
  53-1/RConn2 -- load44/LConn2 -- 44/LConn2
  53-1/RConn3 -- load44/LConn3 -- 44/LConn3
  39/RConn1 -- 53-1/LConn1 -- 54-1/LConn1
  39/RConn2 -- 53-1/LConn2 -- 54-1/LConn2
  39/RConn3 -- 53-1/LConn3 -- 54-1/LConn3
  load39/LConn1 -- Load Flow Bus14/LConn1 -- 39/LConn1
  load39/LConn2 -- 39/LConn2
  load39/LConn3 -- 39/LConn3
  60-1/LConn1 -- 45/RConn1 -- 48-1/LConn1
  60-1/LConn2 -- 45/RConn2 -- 48-1/LConn2
  60-1/LConn3 -- 45/RConn3 -- 48-1/LConn3
  load45/LConn1 -- Load Flow Bus17/LConn1 -- 54-1/RConn1 -- 45/LConn1 -- 59-1/RConn1
  35/LConn1 -- Load Flow Bus11/LConn1 -- 48-1/RConn1
  35/LConn2 -- 48-1/RConn2
  35/LConn3 -- 48-1/RConn3
  A31/RConn1 -- Load Flow Bus7/LConn1 -- 31/LConn1 -- 41-1/RConn1 -- 37-1/RConn1
  B31/RConn1 -- 31/LConn2 -- 41-1/RConn2 -- 37-1/RConn2
  C31/RConn1 -- 31/LConn3 -- 41-1/RConn3 -- 37-1/RConn3
  60-1/RConn1 -- load51/LConn1 -- Load Flow Bus21/LConn1 -- 51/LConn1
  60-1/RConn2 -- load51/LConn2 -- 51/LConn2
  60-1/RConn3 -- 51/LConn3 -- load51/LConn3
  64-1/LConn1 -- 51/RConn1
  64-1/LConn2 -- 51/RConn2
  64-1/LConn3 -- 51/RConn3
  64-1/RConn1 -- load50/LConn1 -- 50/LConn1 -- Load Flow Bus20/LConn1
  50/LConn2 -- load50/LConn2 -- 64-1/RConn2
  50/LConn3 -- load50/LConn3 -- 64-1/RConn3
  50/RConn1 -- a50/RConn1
  50/RConn2 -- b50/RConn1
  50/RConn3 -- c50/RConn1
  61-1/RConn1 -- Load Flow Bus19/LConn1 -- load49/LConn1 -- 49/LConn1
  61-1/RConn2 -- load49/LConn2 -- 49/LConn2
  61-1/RConn3 -- load49/LConn3 -- 49/LConn3
  c49/RConn1 -- 49/RConn3
  b49/RConn1 -- 49/RConn2
  a49/RConn1 -- 49/RConn1
  32/RConn1 -- T32-11/RConn1
  32/RConn2 -- T32-11/RConn2
  32/RConn3 -- T32-11/RConn3
  T32-11/LConn1 -- Load Flow Bus1/LConn1 -- 11/LConn1
  T32-11/LConn2 -- 11/LConn2
  T32-11/LConn3 -- 11/LConn3
  11/RConn2 -- Three-Phase Source1/RConn2 -- G11/LConn2
  11/RConn3 -- Three-Phase Source1/RConn3 -- G11/LConn3
  T13-1/LConn2 -- 13/LConn2
  T13-1/LConn3 -- 13/LConn3
  T34-35/RConn1 -- 35/RConn1
  T34-35/RConn2 -- 35/RConn2
  T34-35/RConn3 -- 35/RConn3
  44-1/LConn3 -- 34/RConn3
  44-1/LConn2 -- 34/RConn2
  44-1/LConn1 -- 34/RConn1
  46/RConn1 -- 52-1/LConn1 -- 61-1/LConn1
  46/RConn2 -- 52-1/LConn2 -- 61-1/LConn2
  52-1/LConn3 -- 46/RConn3 -- 61-1/LConn3
  load46/LConn1 -- Load Flow Bus18/LConn1 -- 46/LConn1
  load46/LConn2 -- 46/LConn2
  load46/LConn3 -- 46/LConn3
  54-1/RConn2 -- load45/LConn2 -- 45/LConn2 -- 59-1/RConn2
  54-1/RConn3 -- 45/LConn3 -- load45/LConn3 -- 59-1/RConn3
  SSN Interface Block (3ph)/RConn1 -- 17-1/LConn1
  SSN Interface Block (3ph)/RConn2 -- 17-1/LConn2
  SSN Interface Block (3ph)/RConn3 -- SSN group tag1/LConn1 -- 17-1/LConn3
  SSN Interface Block (3ph)1/RConn2 -- 52-1/RConn2
  SSN Interface Block (3ph)1/RConn1 -- 52-1/RConn1
  SSN Interface Block (3ph)1/RConn3 -- SSN group tag3/LConn1 -- 52-1/RConn3

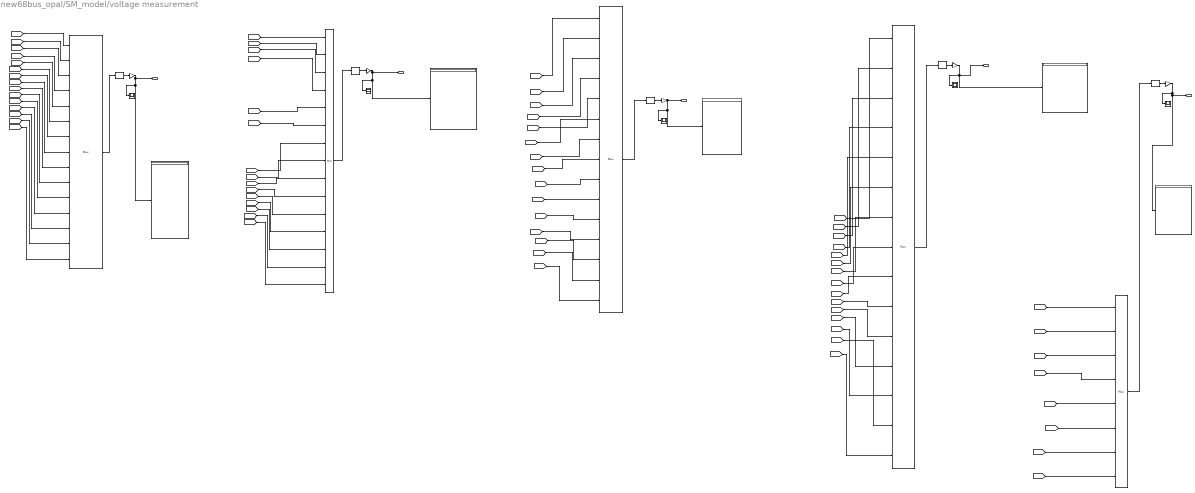
== system new68bus_opal/SM_model/voltage measurement  ==
  Display{,1..4} (5 alike) : Display
  Gain{1..5} (5 alike) : Gain  Gain=sqrt(2)
  Mux{1..4} (4 alike) : Mux  Inputs=15
  Mux5 : Mux  Inputs=8
  RMS{1..5} (5 alike) : powerlib_meascontrol/Measurements/RMS  TrueRMS=on  Freq=60  RMSInit=120  Ts=Ts
      settings: SourceProductName=Simscape Electrical
  Scope{1..5} (5 alike) : Scope
  Output : Outport
  Output1 : Outport  Port=2
  Output2 : Outport  Port=3
  Output3 : Outport  Port=4
  Output4 : Outport  Port=5
  wires:
  Mux1/1 -> RMS2/1
  [Vabc_05] -> Mux1/5
  [Vabc_06] -> Mux1/6
  Gain2/1 -> Output/1, Display/1, Scope1/1
  [Vabc_03] -> Mux1/3
  [Vabc_11] -> Mux1/11
  [Vabc_10] -> Mux1/10
  [Vabc_07] -> Mux1/7
  [Vabc_09] -> Mux1/9
  [Vabc_01] -> Mux1/1
  [Vabc_13] -> Mux1/13
  [Vabc_02] -> Mux1/2
  [Vabc_12] -> Mux1/12
  [Vabc_14] -> Mux1/14
  [Vabc_08] -> Mux1/8
  RMS2/1 -> Gain2/1
  [Vabc_04] -> Mux1/4
  [Vabc_15] -> Mux1/15
  Mux2/1 -> RMS1/1
  RMS1/1 -> Gain1/1
  Gain1/1 -> Scope2/1, Display1/1, Output1/1
  [Vabc_16] -> Mux2/1
  [Vabc_17] -> Mux2/2
  [Vabc_18] -> Mux2/3
  Gain3/1 -> Scope3/1, Display2/1, Output2/1
  RMS3/1 -> Gain3/1
  Mux3/1 -> RMS3/1
  Gain4/1 -> Scope4/1, Output3/1, Display3/1
  RMS4/1 -> Gain4/1
  Mux4/1 -> RMS4/1
  [Vabc_19] -> Mux2/4
  [Vabc_20] -> Mux2/5
  [Vabc_21] -> Mux2/6
  [Vabc_22] -> Mux2/7
  [Vabc_23] -> Mux2/8
  [Vabc_24] -> Mux2/9
  [Vabc_25] -> Mux2/10
  [Vabc_26] -> Mux2/11
  [Vabc_27] -> Mux2/12
  [Vabc_28] -> Mux2/13
  [Vabc_29] -> Mux2/14
  [Vabc_30] -> Mux2/15
  [Vabc_31] -> Mux3/1
  [Vabc_32] -> Mux3/2
  [Vabc_33] -> Mux3/3
  [Vabc_34] -> Mux3/4
  [Vabc_35] -> Mux3/5
  [Vabc_36] -> Mux3/6
  [Vabc_37] -> Mux3/7
  [Vabc_38] -> Mux3/8
  [Vabc_39] -> Mux3/9
  [Vabc_40] -> Mux3/10
  [Vabc_41] -> Mux3/11
  [Vabc_42] -> Mux3/12
  [Vabc_43] -> Mux3/13
  [Vabc_44] -> Mux3/14
  [Vabc_45] -> Mux3/15
  [Vabc_46] -> Mux4/1
  [Vabc_47] -> Mux4/2
  [Vabc_48] -> Mux4/3
  [Vabc_49] -> Mux4/4
  [Vabc_50] -> Mux4/5
  [Vabc_51] -> Mux4/6
  [Vabc_52] -> Mux4/7
  [Vabc_53] -> Mux4/8
  [Vabc_54] -> Mux4/9
  [Vabc_55] -> Mux4/10
  [Vabc_56] -> Mux4/11
  [Vabc_57] -> Mux4/12
  [Vabc_58] -> Mux4/13
  [Vabc_59] -> Mux4/14
  [Vabc_60] -> Mux4/15
  Gain5/1 -> Display4/1, Output4/1, Scope5/1
  RMS5/1 -> Gain5/1
  Mux5/1 -> RMS5/1
  [Vabc_61] -> Mux5/1
  [Vabc_62] -> Mux5/2
  [Vabc_63] -> Mux5/3
  [Vabc_64] -> Mux5/4
  [Vabc_65] -> Mux5/5
  [Vabc_66] -> Mux5/6
  [Vabc_67] -> Mux5/7
  [Vabc_68] -> Mux5/8

== system new68bus_opal/SM_model/Subsystem/G14 ==
  "M14: Turbine & Regulators " : Subsystem
  Pref14 : Constant  Value=0.595
  Vref14 : Constant
  gen14 : powerlib/Machines/Synchronous Machine pu Standard  PresetModel=No  MechanicalLoad=Mechanical power Pm  ShowDetailedParameters=on  RotorType=Round  Units=per unit standard parameters  MeasurementBus=off  NominalParameters="[3000*1e6  13.8e3   60 ]"  Reactances1="[mac_con(14,6:8)  mac_con(14,11:13)  mac_con(14,4)]"  Reactances2=[ 1.305, 0.296, 0.252, 0.474, 0.243, 0.18 ]  dAxisTimeConstants=Open-circuit  qAxisTimeConstants=Open-circuit  TimeConstants1=[]  TimeConstants2="[mac_con(14,9:10)  mac_con(14,14:15)]"  TimeConstants3=[]  TimeConstants4=[]  TimeConstants5=[ 1.01, 0.053, 0.1 ]  TimeConstants6=[]  TimeConstants7=[]  TimeConstants8=[]  StatorResistance=mac_con(14,5)  Mechanical="[ mac_con(14,16)  0  4]"  PolePairs=4  InitialConditions=[0 -76.9944 0.265611 0.265611 0.265611 -15.9627 -135.963 104.037 1.1157]  SetSaturation=off  Saturation=[0.6404,0.7127,0.8441,0.9214,0.9956,1.082,1.19,1.316,1.457;0.7,0.7698,0.8872,0.9466,0.9969,1.046,1.1,1.151,1.201]  LoadFlowParameters=[1 830000000 0 0 0]  TsPowergui=0  TsBlock=-1  IterativeModel=Trapezoidal non iterative  IterativeDiscreteModel=Trapezoidal non iterative  BusType=PV  Pref=1785*1e6  Qref=0  Qmin=-inf  Qmax=inf  PLF=0  QLF=0
      settings: AttributesFormatString=\n\n  SourceProductName=Simscape Electrical
  A : PMIOPort  Side=Left
  B : PMIOPort  Port=2  Side=Left
  C : PMIOPort  Port=3  Side=Left
  wires:
  Vref14/1 -> "M14: Turbine & Regulators "/3(Vref14)
  [PSSmodel] -> "M14: Turbine & Regulators "/4(PSS14)
  gen14/1 -> "M14: Turbine & Regulators "/1(m14)
  "M14: Turbine & Regulators "/2(Vf14) -> gen14/2
  "M14: Turbine & Regulators "/1(Pm14) -> gen14/1
  Pref14/1 -> "M14: Turbine & Regulators "/2(Pref14)
  connections:
  C/RConn1 -- gen14/RConn3
  B/RConn1 -- gen14/RConn2
  A/RConn1 -- gen14/RConn1

== system new68bus_opal/SM_model/Subsystem/G15 ==
  "M15: Turbine & Regulators " : Subsystem
  Pref15 : Constant  Value=0.334
  Vref15 : Constant
  gen15 : powerlib/Machines/Synchronous Machine pu Standard  PresetModel=No  MechanicalLoad=Mechanical power Pm  ShowDetailedParameters=on  RotorType=Round  Units=per unit standard parameters  MeasurementBus=off  NominalParameters="[3000*1e6  13.8e3   60 ]"  Reactances1="[mac_con(15,6:8)  mac_con(15,11:13)  mac_con(15,4)]"  Reactances2=[ 1.305, 0.296, 0.252, 0.474, 0.243, 0.18 ]  dAxisTimeConstants=Open-circuit  qAxisTimeConstants=Open-circuit  TimeConstants1=[]  TimeConstants2="[mac_con(15,9:10)  mac_con(15,14:15)]"  TimeConstants3=[]  TimeConstants4=[]  TimeConstants5=[ 1.01, 0.053, 0.1 ]  TimeConstants6=[]  TimeConstants7=[]  TimeConstants8=[]  StatorResistance=mac_con(15,5)  Mechanical="[ mac_con(15,16)  0  4]"  PolePairs=4  InitialConditions=[0 -76.9944 0.265611 0.265611 0.265611 -15.9627 -135.963 104.037 1.1157]  SetSaturation=off  Saturation=[0.6404,0.7127,0.8441,0.9214,0.9956,1.082,1.19,1.316,1.457;0.7,0.7698,0.8872,0.9466,0.9969,1.046,1.1,1.151,1.201]  LoadFlowParameters=[1 830000000 0 0 0]  TsPowergui=0  TsBlock=-1  IterativeModel=Trapezoidal non iterative  IterativeDiscreteModel=Trapezoidal non iterative  BusType=PV  Pref=1000*1e6  Qref=0  Qmin=-inf  Qmax=inf  PLF=0  QLF=0
      settings: AttributesFormatString=\n\n  SourceProductName=Simscape Electrical
  A : PMIOPort  Side=Left
  B : PMIOPort  Port=2  Side=Left
  C : PMIOPort  Port=3  Side=Left
  wires:
  Pref15/1 -> "M15: Turbine & Regulators "/2(Pref15)
  "M15: Turbine & Regulators "/1(Pm15) -> gen15/1
  "M15: Turbine & Regulators "/2(Vf15) -> gen15/2
  gen15/1 -> "M15: Turbine & Regulators "/1(m15)
  [PSSmodel] -> "M15: Turbine & Regulators "/4(PSS15)
  Vref15/1 -> "M15: Turbine & Regulators "/3(Vref15)
  connections:
  A/RConn1 -- gen15/RConn1
  B/RConn1 -- gen15/RConn2
  C/RConn1 -- gen15/RConn3

== system new68bus_opal/SM_model/Subsystem/G16 ==
  "M16: Turbine & Regulators " : Subsystem
  Pref16 : Constant  Value=0.563
  Vref16 : Constant
  gen16 : powerlib/Machines/Synchronous Machine pu Standard  PresetModel=No  MechanicalLoad=Mechanical power Pm  ShowDetailedParameters=on  RotorType=Round  Units=per unit standard parameters  MeasurementBus=off  NominalParameters="[6000*1e6  13.8e3   60 ]"  Reactances1="[mac_con(16,6:8)  mac_con(16,11:13)  mac_con(16,4)]"  Reactances2=[ 1.305, 0.296, 0.252, 0.474, 0.243, 0.18 ]  dAxisTimeConstants=Open-circuit  qAxisTimeConstants=Open-circuit  TimeConstants1=[]  TimeConstants2="[mac_con(16,9:10)  mac_con(16,14:15)]"  TimeConstants3=[]  TimeConstants4=[]  TimeConstants5=[ 1.01, 0.053, 0.1 ]  TimeConstants6=[]  TimeConstants7=[]  TimeConstants8=[]  StatorResistance=mac_con(16,5)  Mechanical="[ mac_con(16,16)  0  4]"  PolePairs=4  InitialConditions=[0 -63.2657 0.339533 0.339533 0.339533 -35.2425 -155.242 84.7575 1.77729]  SetSaturation=off  Saturation=[0.6404,0.7127,0.8441,0.9214,0.9956,1.082,1.19,1.316,1.457;0.7,0.7698,0.8872,0.9466,0.9969,1.046,1.1,1.151,1.201]  LoadFlowParameters=[1 830000000 0 0 0]  TsPowergui=0  TsBlock=-1  IterativeModel=Trapezoidal non iterative  IterativeDiscreteModel=Trapezoidal non iterative  BusType=swing  Pref=3380*1e6  Qref=0  Qmin=-inf  Qmax=inf  PLF=0  QLF=0
      settings: AttributesFormatString=\n\n  SourceProductName=Simscape Electrical
  A : PMIOPort  Side=Left
  B : PMIOPort  Port=2  Side=Left
  C : PMIOPort  Port=3  Side=Left
  wires:
  Pref16/1 -> "M16: Turbine & Regulators "/2(Pref16)
  "M16: Turbine & Regulators "/1(Pm16) -> gen16/1
  "M16: Turbine & Regulators "/2(Vf16) -> gen16/2
  gen16/1 -> "M16: Turbine & Regulators "/1(m16)
  [PSSmodel] -> "M16: Turbine & Regulators "/4(PSS16)
  Vref16/1 -> "M16: Turbine & Regulators "/3(Vref16)
  connections:
  A/RConn1 -- gen16/RConn1
  B/RConn1 -- gen16/RConn2
  C/RConn1 -- gen16/RConn3
